simulink library "Library"  (R2018a)
settings: Solver=VariableStepAuto  StartTime=0.0  StopTime=10.0  RelTol=1e-3
values from neighbouring files (symbols this model uses):
  alpha = 1e-1*V_m^2    [dVOC.m]
  C_dc = 0.008*(n)    (= 1.6)    [VSM.m]    (also in dVOC.m; droop.m; droop_with_current_limitation.m; matching.m)
  C_f = n*300*10^-6    (= 0.06)    [VSM.m]    (also in dVOC.m; droop.m; droop_with_current_limitation.m; matching.m)
  D_p = (1/(m_p*w_b))    (= 101321.183642)    [VSM.m]
  droop_percentage = 1    [VSM.m]    (also in dVOC.m; droop.m; droop_with_current_limitation.m; matching.m)
  eta = m_p*V_m^2    [dVOC.m]
  eta_1 = w_b/Vdc_n    [VSM.m]    (also in dVOC.m; droop.m; droop_with_current_limitation.m; matching.m)
  i_ll = -1.15*(S_b/Vdc_n)-i_loss_dc    [VSM.m]    (also in dVOC.m; droop.m; droop_with_current_limitation.m; matching.m)
  i_ul = 1.15*(S_b/Vdc_n)+i_loss_dc    [VSM.m]    (also in dVOC.m; droop.m; droop_with_current_limitation.m; matching.m)
  J = D_p*tau_f    (= 2026.42367285)    [VSM.m]
  k_dc = eta_1/(Vdc_n*m_p)    [VSM.m]    (also in dVOC.m; droop.m; droop_with_current_limitation.m; matching.m)
  K_p = (1/Vdc_n)    [VSM.m]    (also in dVOC.m; droop.m; droop_with_current_limitation.m; matching.m)
  K_r = 1/R_dc    [VSM.m]    (also in dVOC.m; droop.m; droop_with_current_limitation.m; matching.m)
  Kff_i = 1    [VSM.m]    (also in dVOC.m; droop.m; droop_with_current_limitation.m; matching.m)
  Kff_v = 1    [VSM.m]    (also in dVOC.m; droop.m; droop_with_current_limitation.m; matching.m)
  Ki_i = (1/n)*1.19    (= 0.00595)    [VSM.m]    (also in dVOC.m; droop.m; droop_with_current_limitation.m; matching.m)
  Ki_v = (n)*1.161022    (= 232.2044)    [VSM.m]    (also in dVOC.m; droop.m; droop_with_current_limitation.m; matching.m)
  ki_v_ac = 4*5.2500e-04    (= 0.0021)    [VSM.m]    (also in dVOC.m = 0.5; droop.m = 0.5; droop_with_current_limitation.m = 0.5; matching.m = 0.5)
  Kp_i = 0.738891    [VSM.m]    (also in dVOC.m; droop.m; droop_with_current_limitation.m; matching.m)
  Kp_v = 0.52    [VSM.m]    (also in dVOC.m; droop.m; droop_with_current_limitation.m; matching.m)
  kp_v_ac = 0.001    [VSM.m]    (also in dVOC.m; droop.m; droop_with_current_limitation.m; matching.m)
  L_f = (1/n)*200*10^-6    (= 1e-06)    [VSM.m]    (also in dVOC.m; droop.m; droop_with_current_limitation.m; matching.m)
  m_p = (2*pi*0.5)/(S_b)    (= 3.14159265359e-08)    [VSM.m]    (also in dVOC.m; droop.m; droop_with_current_limitation.m; matching.m)
  n = 200    [VSM.m]    (also in dVOC.m; droop.m; droop_with_current_limitation.m; matching.m)
  R_dc = (Vdc_n/(0.05*(S_b)/Vdc_n))    [VSM.m]    (also in dVOC.m; droop.m; droop_with_current_limitation.m; matching.m)
  R_f = 0.001/n    (= 5e-06)    [VSM.m]    (also in dVOC.m; droop.m; droop_with_current_limitation.m; matching.m)
  S_b = 100*(10^6)    (= 100000000)    [VSM.m]    (also in dVOC.m; droop.m; droop_with_current_limitation.m; matching.m)
  T_en = T_load-0.5    (= 24.5)    [VSM.m]    (also in dVOC.m; droop.m; droop_with_current_limitation.m; matching.m)
  tau_dc = 0.05    [VSM.m]    (also in dVOC.m; droop.m; droop_with_current_limitation.m; matching.m)
  tau_g = 5    [VSM.m]    (also in dVOC.m; droop.m; droop_with_current_limitation.m; matching.m)
  V2_rms = 13800    [VSM.m]    (also in dVOC.m; droop.m; droop_with_current_limitation.m; matching.m)
  V_m = sqrt(2/3)*V1_rms    [VSM.m]    (also in dVOC.m; droop.m; droop_with_current_limitation.m; matching.m)
  Vdc_n = 3*V_m    [VSM.m]    (also in dVOC.m; droop.m; droop_with_current_limitation.m; matching.m)
  w_b = 2*pi*f_b    (= 314.159265359)    [VSM.m]    (also in dVOC.m; droop.m; droop_with_current_limitation.m; matching.m)
  w_f = 2*pi*5    (= 31.4159265359)    [VSM.m]    (also in dVOC.m; droop.m; droop_with_current_limitation.m; matching.m)
undefined symbols (not defined in the file or in its folder): i_dc, k_v_ac
libraries: powerlib x107, powerlib_meascontrol x48, cstblocks x5, simulink x3, sps_avr x1
(part 1 of 2)
settings Model: Creator=TayyebiA  LastModifiedBy=TayyebiA

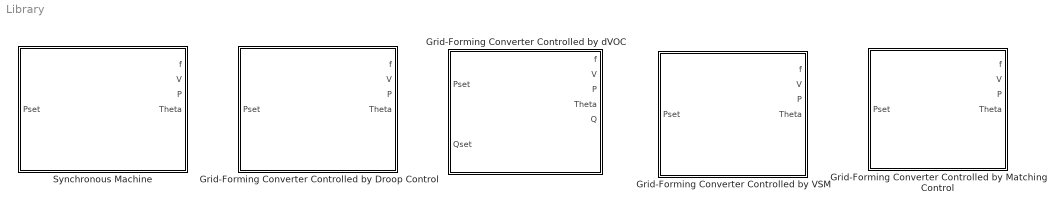
== system Library ==
  "Grid-Forming Converter Controlled by Droop Control " : Subsystem
  Grid-Forming Converter Controlled by Matching Control : Subsystem
  Grid-Forming Converter Controlled by VSM : Subsystem
  "Grid-Forming Converter Controlled by dVOC " : Subsystem
  Synchronous Machine : Subsystem

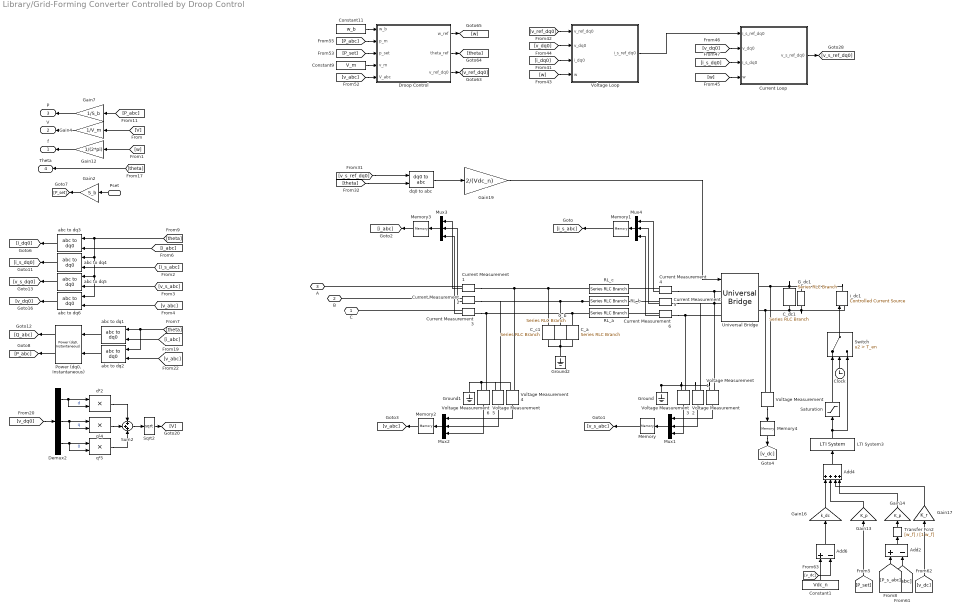
== system Library/Grid-Forming Converter Controlled by Droop Control  ==
  Pset : Inport
  Add2 : Sum  Inputs=+-
  Add4 : Sum  Inputs=++++
  Add6 : Sum  Inputs=+-
  C_a : powerlib/Elements/Series RLC Branch  LConnTagsString=__new0  RConnTagsString=__new0  BranchType=C  Resistance=1  Inductance=1e-3  SetiL0=off  InitialCurrent=0  Capacitance=C_f  Setx0=off  InitialVoltage=165  Measurements=None
  C_b : powerlib/Elements/Series RLC Branch  LConnTagsString=__new0  RConnTagsString=__new0  BranchType=C  Resistance=1  Inductance=1e-3  SetiL0=off  InitialCurrent=0  Capacitance=C_f  Setx0=off  InitialVoltage=165  Measurements=None
  C_c1 : powerlib/Elements/Series RLC Branch  LConnTagsString=__new0  RConnTagsString=__new0  BranchType=C  Resistance=1  Inductance=1e-3  SetiL0=off  InitialCurrent=0  Capacitance=C_f  Setx0=off  InitialVoltage=165  Measurements=None
  C_dc1 : powerlib/Elements/Series RLC Branch  LConnTagsString=__new0  RConnTagsString=__new0  BranchType=C  Resistance=1  Inductance=1e-3  SetiL0=off  InitialCurrent=0  Capacitance=C_dc  Setx0=off  InitialVoltage=Vdc_n  Measurements=None
  Clock : Clock
  Constant1 : Constant  Value=Vdc_n
  Constant11 : Constant  Value=w_b
  Constant9 : Constant  Value=V_m
  Current Loop : Subsystem
  Current Measurement{1..6} (6 alike) : powerlib/Measurements/Current Measurement  PhasorSimulation=off  OutputType=Complex  PSBequivalent=0
  Demux2 : Demux  Outputs=3
  Droop Control : Subsystem
  G_dc1 : powerlib/Elements/Series RLC Branch  LConnTagsString=__new0  RConnTagsString=__new0  BranchType=R  Resistance=R_dc  Inductance=1e-3  SetiL0=off  InitialCurrent=0  Capacitance=1e-6  Setx0=off  InitialVoltage=0  Measurements=None
  Gain12 : Gain  Gain=1/(2*pi)
  Gain13 : Gain  Gain=K_p
  Gain14 : Gain  Gain=K_p
  Gain16 : Gain  Gain=k_dc
  Gain17 : Gain  Gain=K_r
  Gain19 : Gain  Gain=2/(Vdc_n)
  Gain2 : Gain  Gain=S_b
  Gain4 : Gain  Gain=1/V_m
  Gain7 : Gain  Gain=1/S_b
  Ground : powerlib/Elements/Ground  LConnTagsString=a
  Ground1 : powerlib/Elements/Ground  LConnTagsString=a
  Ground2 : powerlib/Elements/Ground  LConnTagsString=a
  LTI System3 : cstblocks/LTI System  sys=tf(1,[tau_dc 1])  IC=[]
  Memory{,1..4} (5 alike) : Memory
  Mux{1..4} (4 alike) : Mux  Inputs=3
  "Power (dq0, Instantaneous)" : powerlib_meascontrol/Measurements/Power (dq0, Instantaneous)
      settings: SourceProductName=Simscape Power Systems  SourceProductBaseCode=PS
  RL_a : powerlib/Elements/Series RLC Branch  LConnTagsString=__new0  RConnTagsString=__new0  BranchType=RL  Resistance=R_f  Inductance=L_f  SetiL0=off  InitialCurrent=0  Capacitance=1e-6  Setx0=off  InitialVoltage=0  Measurements=Branch voltage and current
  RL_b : powerlib/Elements/Series RLC Branch  LConnTagsString=__new0  RConnTagsString=__new0  BranchType=RL  Resistance=R_f  Inductance=L_f  SetiL0=off  InitialCurrent=0  Capacitance=1e-6  Setx0=off  InitialVoltage=0  Measurements=None
  RL_c : powerlib/Elements/Series RLC Branch  LConnTagsString=__new0  RConnTagsString=__new0  BranchType=RL  Resistance=R_f  Inductance=L_f  SetiL0=off  InitialCurrent=0  Capacitance=1e-6  Setx0=off  InitialVoltage=0  Measurements=None
  Saturation : Saturate  UpperLimit=i_ul  LowerLimit=i_ll
  Sqrt2 : Sqrt  SaturateOnIntegerOverflow=on
  Sum2 : Sum  Inputs=+++  SaturateOnIntegerOverflow=on  InputSameDT=on  OutDataTypeStr=Inherit: Same as first input
  Switch : Switch  Criteria=u2 > Threshold  Threshold=T_en
  Transfer Fcn2 : TransferFcn  Numerator=[w_f]  Denominator=[1 w_f]
  Universal Bridge : powerlib/Power Electronics/Universal Bridge  Arms=3  SnubberResistance=1e5  SnubberCapacitance=inf  Device=Average-model based VSC  Ron=1e-3  Lon=0  ForwardVoltages="[  0  0  ]"  ForwardVoltage=0  GTOparameters=[ 10e-6 , 20e-6 ]  IGBTparameters=[ 1e-6 , 2e-6 ]  Measurements=None  Measurements_2=None  converterType=Rectifier
  Voltage Loop : Subsystem
  Voltage Measurement{,1..6} (7 alike) : powerlib/Measurements/Voltage Measurement  PhasorSimulation=off  OutputType=Complex  PSBequivalent=0
  abc to dq{1..6} (6 alike) : powerlib_meascontrol/Transformations/abc to dq0  Alignment=90 degrees behind phase A axis
  dq0 to abc : powerlib_meascontrol/Transformations/dq0 to abc  Alignment=90 degrees behind phase A axis
  d²2 : Product  SaturateOnIntegerOverflow=on  RndMeth=Zero  InputSameDT=on  OutDataTypeStr=Inherit: Same as first input
  i_dc1 : powerlib/Electrical Sources/Controlled Current Source  Initialize=off  Source_Type=DC  Amplitude=i_dc  Phase=0  Frequency=0  Measurements=None
  q²4 : Product  SaturateOnIntegerOverflow=on  RndMeth=Zero  InputSameDT=on  OutDataTypeStr=Inherit: Same as first input
  q²5 : Product  SaturateOnIntegerOverflow=on  RndMeth=Zero  InputSameDT=on  OutDataTypeStr=Inherit: Same as first input
  C : PMIOPort  Side=Right
  B : PMIOPort  Port=2  Side=Right
  A : PMIOPort  Port=3  Side=Right
  f : Outport
  V : Outport  Port=2
  P : Outport  Port=3
  Theta : Outport  Port=4
  wires:
  Add4/1 -> LTI System3/1
  Clock/1 -> Switch/2
  Saturation/1 -> Switch/1
  LTI System3/1 -> Switch/3, Saturation/1
  Gain7/1 -> P/1
  [P_abc] -> Gain7/1
  Current Measurement6/1 -> Mux4/3
  Current Measurement5/1 -> Mux4/2
  Current Measurement4/1 -> Mux4/1
  Current Measurement3/1 -> Mux3/3
  Current Measurement2/1 -> Mux3/2
  Current Measurement1/1 -> Mux3/1
  Voltage Measurement4/1 -> Mux2/1
  Voltage Measurement5/1 -> Mux2/2
  Voltage Measurement6/1 -> Mux2/3
  Voltage Measurement3/1 -> Mux1/3
  Voltage Measurement2/1 -> Mux1/2
  Voltage Measurement1/1 -> Mux1/1
  [V] -> Gain4/1
  Gain2/1 -> [P_set]
  Pset/1 -> Gain2/1
  Gain12/1 -> f/1
  [w] -> Gain12/1
  Mux2/1 -> Memory2/1
  Mux3/1 -> Memory3/1
  Mux1/1 -> Memory/1
  abc to dq1/1 -> "Power (dq0, Instantaneous)"/2
  abc to dq2/1 -> "Power (dq0, Instantaneous)"/1
  [theta] -> abc to dq2/2, abc to dq1/2
  [v_abc] -> abc to dq2/1
  "Power (dq0, Instantaneous)"/2 -> [Q_abc]
  "Power (dq0, Instantaneous)"/1 -> [P_abc]
  [i_abc] -> abc to dq1/1
  Gain4/1 -> V/1
  [theta] -> Theta/1
  [i_abc] -> abc to dq3/1
  [i_s_abc] -> abc to dq4/1
  [v_abc] -> abc to dq6/1
  [v_s_abc] -> abc to dq5/1
  [theta] -> abc to dq4/2, abc to dq5/2, abc to dq6/2, abc to dq3/2
  abc to dq3/1 -> [i_dq0]
  abc to dq4/1 -> [i_s_dq0]
  abc to dq5/1 -> [v_s_dq0]
  abc to dq6/1 -> [v_dq0]
  [theta] -> dq0 to abc/2
  q²4/1 -> Sum2/2
  [v_dq0] -> Demux2/1
  q²5/1 -> Sum2/3
  Sum2/1 -> Sqrt2/1
  Demux2/3 -> q²5/1, q²5/2  "0"
  d²2/1 -> Sum2/1
  Demux2/2 -> q²4/1, q²4/2  "q"
  Demux2/1 -> d²2/1, d²2/2  "d"
  Sqrt2/1 -> [V]
  Mux4/1 -> Memory1/1
  Memory2/1 -> [v_abc]
  Memory3/1 -> [i_abc]
  Voltage Measurement/1 -> Memory4/1
  Memory4/1 -> [v_dc]
  Memory/1 -> [v_s_abc]
  Memory1/1 -> [i_s_abc]
  dq0 to abc/1 -> Gain19/1
  [w] -> Current Loop/4(w)
  [v_ref_dq0] -> Voltage Loop/1(v_ref_dq0)
  [i_dq0] -> Voltage Loop/3(i_dq0)
  Voltage Loop/1(i_s_ref_dq0) -> Current Loop/1(i_s_ref_dq0)
  [v_dq0] -> Current Loop/2(v_dq0)
  [i_s_dq0] -> Current Loop/3(i_s_dq0)
  Current Loop/1(v_s_ref_dq0) -> [v_s_ref_dq0]
  [w] -> Voltage Loop/4(w)
  [v_dq0] -> Voltage Loop/2(v_dq0)
  Switch/1 -> i_dc1/1
  Gain19/1 -> Universal Bridge/1
  [v_s_ref_dq0] -> dq0 to abc/1
  Constant11/1 -> Droop Control/1(w_b)
  Droop Control/3(v_ref_dq0) -> [v_ref_dq0]
  [P_abc] -> Droop Control/2(p_m)
  Constant9/1 -> Droop Control/4(v_m)
  [v_abc] -> Droop Control/5(V_abc)
  Droop Control/2(theta_ref) -> [theta]
  Droop Control/1(w_ref) -> [w]
  [P_set] -> Droop Control/3(p_set)
  [P_abc] -> Add2/2
  Gain14/1 -> Add4/4
  [P_set] -> Gain13/1
  Gain13/1 -> Add4/2
  Gain16/1 -> Add4/1
  Constant1/1 -> Add6/1
  Gain17/1 -> Add4/3
  Add2/1 -> Transfer Fcn2/1
  Transfer Fcn2/1 -> Gain14/1
  [v_dc] -> Add6/2
  Add6/1 -> Gain16/1
  [P_s_abc] -> Add2/1
  [v_dc] -> Gain17/1
  connections:
  RL_b/RConn1 -- Voltage Measurement5/LConn1 -- Current Measurement2/LConn1 -- C_b/LConn1
  Voltage Measurement6/LConn1 -- Current Measurement3/LConn1 -- C_a/LConn1 -- RL_a/RConn1
  Current Measurement4/RConn1 -- RL_c/LConn1
  Current Measurement6/RConn1 -- RL_a/LConn1
  Current Measurement5/RConn1 -- RL_b/LConn1
  Voltage Measurement/LConn1 -- Universal Bridge/RConn1 -- C_dc1/LConn1 -- G_dc1/LConn1 -- i_dc1/RConn1
  Voltage Measurement6/LConn2 -- Voltage Measurement5/LConn2 -- Voltage Measurement4/LConn2 -- Ground1/LConn1
  Ground/LConn1 -- Voltage Measurement2/LConn2 -- Voltage Measurement1/LConn2 -- Voltage Measurement3/LConn2
  Current Measurement3/RConn1 -- C/RConn1
  Current Measurement2/RConn1 -- B/RConn1
  Current Measurement1/RConn1 -- A/RConn1
  Current Measurement6/LConn1 -- Universal Bridge/LConn3 -- Voltage Measurement3/LConn1
  Universal Bridge/LConn2 -- Current Measurement5/LConn1 -- Voltage Measurement2/LConn1
  Universal Bridge/LConn1 -- Current Measurement4/LConn1 -- Voltage Measurement1/LConn1
  Universal Bridge/RConn2 -- Voltage Measurement/LConn2 -- C_dc1/RConn1 -- G_dc1/RConn1 -- i_dc1/LConn1
  C_b/RConn1 -- C_a/RConn1 -- Ground2/LConn1 -- C_c1/RConn1
  Voltage Measurement4/LConn1 -- Current Measurement1/LConn1 -- C_c1/LConn1 -- RL_c/RConn1

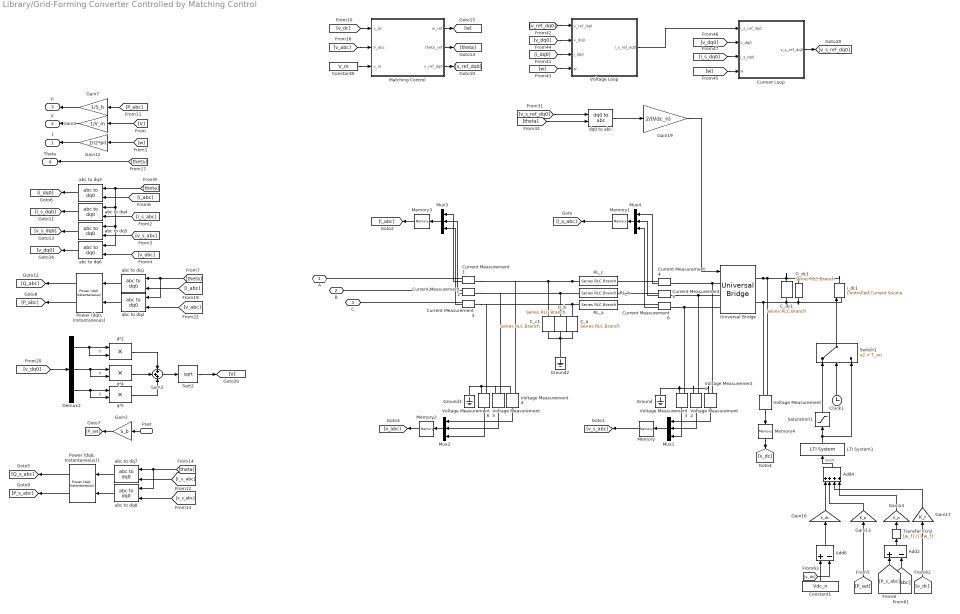
== system Library/Grid-Forming Converter Controlled by Matching Control ==
  Pset : Inport
  Add2 : Sum  Inputs=+-
  Add4 : Sum  Inputs=++++
  Add6 : Sum  Inputs=+-
  C_a : powerlib/Elements/Series RLC Branch  LConnTagsString=__new0  RConnTagsString=__new0  BranchType=C  Resistance=1  Inductance=1e-3  SetiL0=off  InitialCurrent=0  Capacitance=C_f  Setx0=off  InitialVoltage=165  Measurements=None
  C_b : powerlib/Elements/Series RLC Branch  LConnTagsString=__new0  RConnTagsString=__new0  BranchType=C  Resistance=1  Inductance=1e-3  SetiL0=off  InitialCurrent=0  Capacitance=C_f  Setx0=off  InitialVoltage=165  Measurements=None
  C_c1 : powerlib/Elements/Series RLC Branch  LConnTagsString=__new0  RConnTagsString=__new0  BranchType=C  Resistance=1  Inductance=1e-3  SetiL0=off  InitialCurrent=0  Capacitance=C_f  Setx0=off  InitialVoltage=165  Measurements=None
  C_dc1 : powerlib/Elements/Series RLC Branch  LConnTagsString=__new0  RConnTagsString=__new0  BranchType=C  Resistance=1  Inductance=1e-3  SetiL0=off  InitialCurrent=0  Capacitance=C_dc  Setx0=off  InitialVoltage=Vdc_n  Measurements=None
  Clock1 : Clock
  Constant1 : Constant  Value=Vdc_n
  Constant8 : Constant  Value=V_m
  Current Loop : Subsystem
  Current Measurement{1..6} (6 alike) : powerlib/Measurements/Current Measurement  PhasorSimulation=off  OutputType=Complex  PSBequivalent=0
  Demux2 : Demux  Outputs=3
  G_dc1 : powerlib/Elements/Series RLC Branch  LConnTagsString=__new0  RConnTagsString=__new0  BranchType=R  Resistance=R_dc  Inductance=1e-3  SetiL0=off  InitialCurrent=0  Capacitance=1e-6  Setx0=off  InitialVoltage=0  Measurements=None
  Gain12 : Gain  Gain=1/(2*pi)
  Gain13 : Gain  Gain=K_p
  Gain14 : Gain  Gain=K_p
  Gain16 : Gain  Gain=k_dc
  Gain17 : Gain  Gain=K_r
  Gain19 : Gain  Gain=2/(Vdc_n)
  Gain2 : Gain  Gain=S_b
  Gain4 : Gain  Gain=1/V_m
  Gain7 : Gain  Gain=1/S_b
  Ground : powerlib/Elements/Ground  LConnTagsString=a
  Ground1 : powerlib/Elements/Ground  LConnTagsString=a
  Ground2 : powerlib/Elements/Ground  LConnTagsString=a
  LTI System1 : cstblocks/LTI System  sys=tf(1,[tau_dc 1])  IC=[]
  Matching Control : Subsystem
  Memory{,1..4} (5 alike) : Memory
  Mux{1..4} (4 alike) : Mux  Inputs=3
  "Power (dq0, Instantaneous)" : powerlib_meascontrol/Measurements/Power (dq0, Instantaneous)
      settings: SourceProductName=Simscape Power Systems  SourceProductBaseCode=PS
  "Power (dq0, Instantaneous)1" : powerlib_meascontrol/Measurements/Power (dq0, Instantaneous)
      settings: SourceProductName=Simscape Power Systems  SourceProductBaseCode=PS
  RL_a : powerlib/Elements/Series RLC Branch  LConnTagsString=__new0  RConnTagsString=__new0  BranchType=RL  Resistance=R_f  Inductance=L_f  SetiL0=off  InitialCurrent=0  Capacitance=1e-6  Setx0=off  InitialVoltage=0  Measurements=Branch voltage and current
  RL_b : powerlib/Elements/Series RLC Branch  LConnTagsString=__new0  RConnTagsString=__new0  BranchType=RL  Resistance=R_f  Inductance=L_f  SetiL0=off  InitialCurrent=0  Capacitance=1e-6  Setx0=off  InitialVoltage=0  Measurements=None
  RL_c : powerlib/Elements/Series RLC Branch  LConnTagsString=__new0  RConnTagsString=__new0  BranchType=RL  Resistance=R_f  Inductance=L_f  SetiL0=off  InitialCurrent=0  Capacitance=1e-6  Setx0=off  InitialVoltage=0  Measurements=None
  Saturation1 : Saturate  UpperLimit=i_ul  LowerLimit=i_ll
  Sqrt2 : Sqrt  SaturateOnIntegerOverflow=on
  Sum2 : Sum  Inputs=+++  SaturateOnIntegerOverflow=on  InputSameDT=on  OutDataTypeStr=Inherit: Same as first input
  Switch1 : Switch  Criteria=u2 > Threshold  Threshold=T_en
  Transfer Fcn2 : TransferFcn  Numerator=[w_f]  Denominator=[1 w_f]
  Universal Bridge : powerlib/Power Electronics/Universal Bridge  Arms=3  SnubberResistance=1e5  SnubberCapacitance=inf  Device=Average-model based VSC  Ron=1e-3  Lon=0  ForwardVoltages="[  0  0  ]"  ForwardVoltage=0  GTOparameters=[ 10e-6 , 20e-6 ]  IGBTparameters=[ 1e-6 , 2e-6 ]  Measurements=None  Measurements_2=None  converterType=Rectifier
  Voltage Loop : Subsystem
  Voltage Measurement{,1..6} (7 alike) : powerlib/Measurements/Voltage Measurement  PhasorSimulation=off  OutputType=Complex  PSBequivalent=0
  abc to dq{1..8} (8 alike) : powerlib_meascontrol/Transformations/abc to dq0  Alignment=90 degrees behind phase A axis
  dq0 to abc : powerlib_meascontrol/Transformations/dq0 to abc  Alignment=90 degrees behind phase A axis
  d²2 : Product  SaturateOnIntegerOverflow=on  RndMeth=Zero  InputSameDT=on  OutDataTypeStr=Inherit: Same as first input
  i_dc1 : powerlib/Electrical Sources/Controlled Current Source  Initialize=off  Source_Type=DC  Amplitude=i_dc  Phase=0  Frequency=0  Measurements=None
  q²4 : Product  SaturateOnIntegerOverflow=on  RndMeth=Zero  InputSameDT=on  OutDataTypeStr=Inherit: Same as first input
  q²5 : Product  SaturateOnIntegerOverflow=on  RndMeth=Zero  InputSameDT=on  OutDataTypeStr=Inherit: Same as first input
  A : PMIOPort  Side=Right
  B : PMIOPort  Port=2  Side=Right
  C : PMIOPort  Port=3  Side=Right
  f : Outport
  V : Outport  Port=2
  P : Outport  Port=3
  Theta : Outport  Port=4
  wires:
  [v_s_ref_dq0] -> dq0 to abc/1
  Gain19/1 -> Universal Bridge/1
  Switch1/1 -> i_dc1/1
  [v_dq0] -> Voltage Loop/2(v_dq0)
  [w] -> Voltage Loop/4(w)
  Current Loop/1(v_s_ref_dq0) -> [v_s_ref_dq0]
  [i_s_dq0] -> Current Loop/3(i_s_dq0)
  [v_dq0] -> Current Loop/2(v_dq0)
  Voltage Loop/1(i_s_ref_dq0) -> Current Loop/1(i_s_ref_dq0)
  [i_dq0] -> Voltage Loop/3(i_dq0)
  [v_ref_dq0] -> Voltage Loop/1(v_ref_dq0)
  [w] -> Current Loop/4(w)
  dq0 to abc/1 -> Gain19/1
  Memory1/1 -> [i_s_abc]
  Memory/1 -> [v_s_abc]
  Memory4/1 -> [v_dc]
  Voltage Measurement/1 -> Memory4/1
  Memory3/1 -> [i_abc]
  Memory2/1 -> [v_abc]
  Mux4/1 -> Memory1/1
  Sqrt2/1 -> [V]
  Demux2/1 -> d²2/2, d²2/1  "d"
  Demux2/2 -> q²4/2, q²4/1  "q"
  d²2/1 -> Sum2/1
  Demux2/3 -> q²5/2, q²5/1  "0"
  Sum2/1 -> Sqrt2/1
  q²5/1 -> Sum2/3
  [v_dq0] -> Demux2/1
  q²4/1 -> Sum2/2
  [theta] -> dq0 to abc/2
  abc to dq6/1 -> [v_dq0]
  abc to dq5/1 -> [v_s_dq0]
  abc to dq4/1 -> [i_s_dq0]
  abc to dq3/1 -> [i_dq0]
  [theta] -> abc to dq3/2, abc to dq6/2, abc to dq5/2, abc to dq4/2
  [v_s_abc] -> abc to dq5/1
  [v_abc] -> abc to dq6/1
  [i_s_abc] -> abc to dq4/1
  [i_abc] -> abc to dq3/1
  [theta] -> Theta/1
  Gain4/1 -> V/1
  [i_abc] -> abc to dq1/1
  "Power (dq0, Instantaneous)"/1 -> [P_abc]
  "Power (dq0, Instantaneous)"/2 -> [Q_abc]
  [v_abc] -> abc to dq2/1
  [theta] -> abc to dq1/2, abc to dq2/2
  abc to dq2/1 -> "Power (dq0, Instantaneous)"/1
  abc to dq1/1 -> "Power (dq0, Instantaneous)"/2
  Mux1/1 -> Memory/1
  Mux3/1 -> Memory3/1
  Mux2/1 -> Memory2/1
  [w] -> Gain12/1
  Gain12/1 -> f/1
  Pset/1 -> Gain2/1
  Gain2/1 -> [P_set]
  [V] -> Gain4/1
  Voltage Measurement1/1 -> Mux1/1
  Voltage Measurement2/1 -> Mux1/2
  Voltage Measurement3/1 -> Mux1/3
  Voltage Measurement6/1 -> Mux2/3
  Voltage Measurement5/1 -> Mux2/2
  Voltage Measurement4/1 -> Mux2/1
  Current Measurement1/1 -> Mux3/1
  Current Measurement2/1 -> Mux3/2
  Current Measurement3/1 -> Mux3/3
  Current Measurement4/1 -> Mux4/1
  Current Measurement5/1 -> Mux4/2
  Current Measurement6/1 -> Mux4/3
  [P_abc] -> Gain7/1
  Gain7/1 -> P/1
  [P_s_abc] -> Add2/1
  [v_dc] -> Gain17/1
  Gain17/1 -> Add4/3
  Constant1/1 -> Add6/1
  Clock1/1 -> Switch1/2
  [P_abc] -> Add2/2
  Add6/1 -> Gain16/1
  Add4/1 -> LTI System1/1  "input"
  [P_set] -> Gain13/1
  Gain14/1 -> Add4/4
  Saturation1/1 -> Switch1/1
  LTI System1/1 -> Saturation1/1, Switch1/3
  Gain16/1 -> Add4/1
  Constant8/1 -> Matching Control/3(v_m)
  Matching Control/3(v_ref_dq0) -> [v_ref_dq0]
  Matching Control/2(theta_ref) -> [theta]
  Gain13/1 -> Add4/2
  [v_dc] -> Matching Control/1(v_dc)
  [v_dc] -> Add6/2
  [v_abc] -> Matching Control/2(V_abc)
  Transfer Fcn2/1 -> Gain14/1
  Matching Control/1(w_ref) -> [w]
  Add2/1 -> Transfer Fcn2/1
  abc to dq8/1 -> "Power (dq0, Instantaneous)1"/1
  [i_s_abc] -> abc to dq7/1
  [v_s_abc] -> abc to dq8/1
  abc to dq7/1 -> "Power (dq0, Instantaneous)1"/2
  [theta] -> abc to dq7/2, abc to dq8/2
  "Power (dq0, Instantaneous)1"/2 -> [Q_s_abc]
  "Power (dq0, Instantaneous)1"/1 -> [P_s_abc]
  connections:
  RL_c/RConn1 -- C_c1/LConn1 -- Current Measurement1/LConn1 -- Voltage Measurement4/LConn1
  C_c1/RConn1 -- Ground2/LConn1 -- C_a/RConn1 -- C_b/RConn1
  Universal Bridge/RConn2 -- i_dc1/LConn1 -- G_dc1/RConn1 -- C_dc1/RConn1 -- Voltage Measurement/LConn2
  Voltage Measurement1/LConn1 -- Current Measurement4/LConn1 -- Universal Bridge/LConn1
  Voltage Measurement2/LConn1 -- Current Measurement5/LConn1 -- Universal Bridge/LConn2
  Voltage Measurement3/LConn1 -- Universal Bridge/LConn3 -- Current Measurement6/LConn1
  Current Measurement1/RConn1 -- A/RConn1
  Current Measurement2/RConn1 -- B/RConn1
  Current Measurement3/RConn1 -- C/RConn1
  Voltage Measurement3/LConn2 -- Voltage Measurement1/LConn2 -- Voltage Measurement2/LConn2 -- Ground/LConn1
  Ground1/LConn1 -- Voltage Measurement4/LConn2 -- Voltage Measurement5/LConn2 -- Voltage Measurement6/LConn2
  Universal Bridge/RConn1 -- Voltage Measurement/LConn1 -- i_dc1/RConn1 -- G_dc1/LConn1 -- C_dc1/LConn1
  Current Measurement5/RConn1 -- RL_b/LConn1
  Current Measurement6/RConn1 -- RL_a/LConn1
  Current Measurement4/RConn1 -- RL_c/LConn1
  RL_a/RConn1 -- C_a/LConn1 -- Current Measurement3/LConn1 -- Voltage Measurement6/LConn1
  C_b/LConn1 -- Current Measurement2/LConn1 -- Voltage Measurement5/LConn1 -- RL_b/RConn1

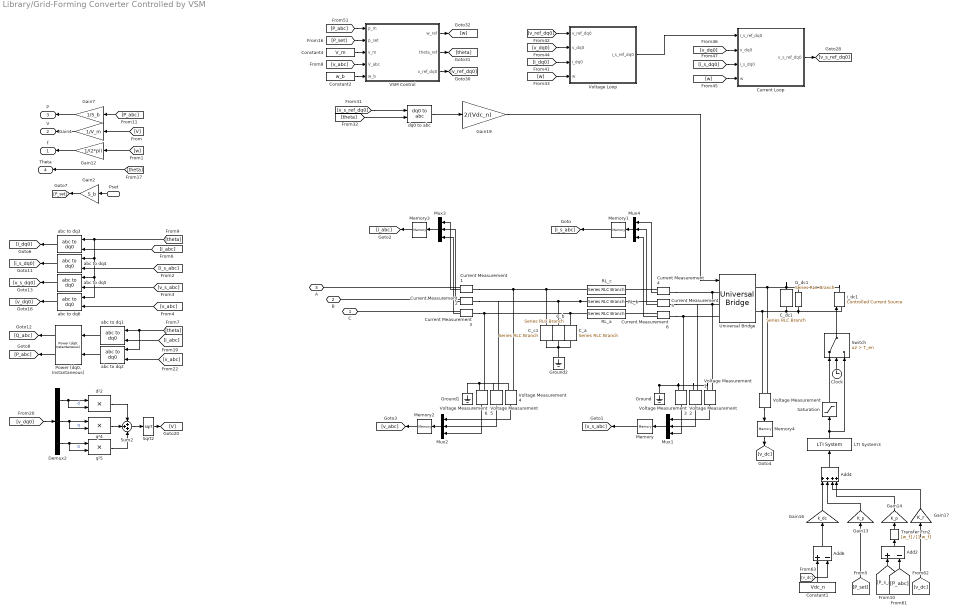
== system Library/Grid-Forming Converter Controlled by VSM ==
  Pset : Inport
  Add2 : Sum  Inputs=+-
  Add4 : Sum  Inputs=++++
  Add6 : Sum  Inputs=+-
  C_a : powerlib/Elements/Series RLC Branch  LConnTagsString=__new0  RConnTagsString=__new0  BranchType=C  Resistance=1  Inductance=1e-3  SetiL0=off  InitialCurrent=0  Capacitance=C_f  Setx0=off  InitialVoltage=165  Measurements=None
  C_b : powerlib/Elements/Series RLC Branch  LConnTagsString=__new0  RConnTagsString=__new0  BranchType=C  Resistance=1  Inductance=1e-3  SetiL0=off  InitialCurrent=0  Capacitance=C_f  Setx0=off  InitialVoltage=165  Measurements=None
  C_c1 : powerlib/Elements/Series RLC Branch  LConnTagsString=__new0  RConnTagsString=__new0  BranchType=C  Resistance=1  Inductance=1e-3  SetiL0=off  InitialCurrent=0  Capacitance=C_f  Setx0=off  InitialVoltage=165  Measurements=None
  C_dc1 : powerlib/Elements/Series RLC Branch  LConnTagsString=__new0  RConnTagsString=__new0  BranchType=C  Resistance=1  Inductance=1e-3  SetiL0=off  InitialCurrent=0  Capacitance=C_dc  Setx0=off  InitialVoltage=Vdc_n  Measurements=None
  Clock : Clock
  Constant1 : Constant  Value=Vdc_n
  Constant2 : Constant  Value=w_b
  Constant4 : Constant  Value=V_m
  Current Loop : Subsystem
  Current Measurement{1..6} (6 alike) : powerlib/Measurements/Current Measurement  PhasorSimulation=off  OutputType=Complex  PSBequivalent=0
  Demux2 : Demux  Outputs=3
  G_dc1 : powerlib/Elements/Series RLC Branch  LConnTagsString=__new0  RConnTagsString=__new0  BranchType=R  Resistance=R_dc  Inductance=1e-3  SetiL0=off  InitialCurrent=0  Capacitance=1e-6  Setx0=off  InitialVoltage=0  Measurements=None
  Gain12 : Gain  Gain=1/(2*pi)
  Gain13 : Gain  Gain=K_p
  Gain14 : Gain  Gain=K_p
  Gain16 : Gain  Gain=k_dc
  Gain17 : Gain  Gain=K_r
  Gain19 : Gain  Gain=2/(Vdc_n)
  Gain2 : Gain  Gain=S_b
  Gain4 : Gain  Gain=1/V_m
  Gain7 : Gain  Gain=1/S_b
  Ground : powerlib/Elements/Ground  LConnTagsString=a
  Ground1 : powerlib/Elements/Ground  LConnTagsString=a
  Ground2 : powerlib/Elements/Ground  LConnTagsString=a
  LTI System3 : cstblocks/LTI System  sys=tf(1,[tau_dc 1])  IC=[]
  Memory{,1..4} (5 alike) : Memory
  Mux{1..4} (4 alike) : Mux  Inputs=3
  "Power (dq0, Instantaneous)" : powerlib_meascontrol/Measurements/Power (dq0, Instantaneous)
      settings: SourceProductName=Simscape Power Systems  SourceProductBaseCode=PS
  RL_a : powerlib/Elements/Series RLC Branch  LConnTagsString=__new0  RConnTagsString=__new0  BranchType=RL  Resistance=R_f  Inductance=L_f  SetiL0=off  InitialCurrent=0  Capacitance=1e-6  Setx0=off  InitialVoltage=0  Measurements=Branch voltage and current
  RL_b : powerlib/Elements/Series RLC Branch  LConnTagsString=__new0  RConnTagsString=__new0  BranchType=RL  Resistance=R_f  Inductance=L_f  SetiL0=off  InitialCurrent=0  Capacitance=1e-6  Setx0=off  InitialVoltage=0  Measurements=None
  RL_c : powerlib/Elements/Series RLC Branch  LConnTagsString=__new0  RConnTagsString=__new0  BranchType=RL  Resistance=R_f  Inductance=L_f  SetiL0=off  InitialCurrent=0  Capacitance=1e-6  Setx0=off  InitialVoltage=0  Measurements=None
  Saturation : Saturate  UpperLimit=i_ul  LowerLimit=i_ll
  Sqrt2 : Sqrt  SaturateOnIntegerOverflow=on
  Sum2 : Sum  Inputs=+++  SaturateOnIntegerOverflow=on  InputSameDT=on  OutDataTypeStr=Inherit: Same as first input
  Switch : Switch  Criteria=u2 > Threshold  Threshold=T_en
  Transfer Fcn2 : TransferFcn  Numerator=[w_f]  Denominator=[1 w_f]
  Universal Bridge : powerlib/Power Electronics/Universal Bridge  Arms=3  SnubberResistance=1e5  SnubberCapacitance=inf  Device=Average-model based VSC  Ron=1e-3  Lon=0  ForwardVoltages="[  0  0  ]"  ForwardVoltage=0  GTOparameters=[ 10e-6 , 20e-6 ]  IGBTparameters=[ 1e-6 , 2e-6 ]  Measurements=None  Measurements_2=None  converterType=Rectifier
  VSM Control : Subsystem
  Voltage Loop : Subsystem
  Voltage Measurement{,1..6} (7 alike) : powerlib/Measurements/Voltage Measurement  PhasorSimulation=off  OutputType=Complex  PSBequivalent=0
  abc to dq{1..6} (6 alike) : powerlib_meascontrol/Transformations/abc to dq0  Alignment=90 degrees behind phase A axis
  dq0 to abc : powerlib_meascontrol/Transformations/dq0 to abc  Alignment=90 degrees behind phase A axis
  d²2 : Product  SaturateOnIntegerOverflow=on  RndMeth=Zero  InputSameDT=on  OutDataTypeStr=Inherit: Same as first input
  i_dc1 : powerlib/Electrical Sources/Controlled Current Source  Initialize=off  Source_Type=DC  Amplitude=i_dc  Phase=0  Frequency=0  Measurements=None
  q²4 : Product  SaturateOnIntegerOverflow=on  RndMeth=Zero  InputSameDT=on  OutDataTypeStr=Inherit: Same as first input
  q²5 : Product  SaturateOnIntegerOverflow=on  RndMeth=Zero  InputSameDT=on  OutDataTypeStr=Inherit: Same as first input
  C : PMIOPort  Side=Right
  B : PMIOPort  Port=2  Side=Right
  A : PMIOPort  Port=3  Side=Right
  f : Outport
  V : Outport  Port=2
  P : Outport  Port=3
  Theta : Outport  Port=4
  wires:
  Add4/1 -> LTI System3/1
  Clock/1 -> Switch/2
  Saturation/1 -> Switch/1
  LTI System3/1 -> Switch/3, Saturation/1
  Gain7/1 -> P/1
  [P_abc] -> Gain7/1
  Current Measurement6/1 -> Mux4/3
  Current Measurement5/1 -> Mux4/2
  Current Measurement4/1 -> Mux4/1
  Current Measurement3/1 -> Mux3/3
  Current Measurement2/1 -> Mux3/2
  Current Measurement1/1 -> Mux3/1
  Voltage Measurement4/1 -> Mux2/1
  Voltage Measurement5/1 -> Mux2/2
  Voltage Measurement6/1 -> Mux2/3
  Voltage Measurement3/1 -> Mux1/3
  Voltage Measurement2/1 -> Mux1/2
  Voltage Measurement1/1 -> Mux1/1
  [V] -> Gain4/1
  Gain2/1 -> [P_set]
  Pset/1 -> Gain2/1
  Gain12/1 -> f/1
  [w] -> Gain12/1
  Mux2/1 -> Memory2/1
  Mux3/1 -> Memory3/1
  Mux1/1 -> Memory/1
  abc to dq1/1 -> "Power (dq0, Instantaneous)"/2
  abc to dq2/1 -> "Power (dq0, Instantaneous)"/1
  [theta] -> abc to dq2/2, abc to dq1/2
  [v_abc] -> abc to dq2/1
  "Power (dq0, Instantaneous)"/2 -> [Q_abc]
  "Power (dq0, Instantaneous)"/1 -> [P_abc]
  [i_abc] -> abc to dq1/1
  Gain4/1 -> V/1
  [theta] -> Theta/1
  [i_abc] -> abc to dq3/1
  [i_s_abc] -> abc to dq4/1
  [v_abc] -> abc to dq6/1
  [v_s_abc] -> abc to dq5/1
  [theta] -> abc to dq4/2, abc to dq5/2, abc to dq6/2, abc to dq3/2
  abc to dq3/1 -> [i_dq0]
  abc to dq4/1 -> [i_s_dq0]
  abc to dq5/1 -> [v_s_dq0]
  abc to dq6/1 -> [v_dq0]
  [theta] -> dq0 to abc/2
  q²4/1 -> Sum2/2
  [v_dq0] -> Demux2/1
  q²5/1 -> Sum2/3
  Sum2/1 -> Sqrt2/1
  Demux2/3 -> q²5/1, q²5/2  "0"
  d²2/1 -> Sum2/1
  Demux2/2 -> q²4/1, q²4/2  "q"
  Demux2/1 -> d²2/1, d²2/2  "d"
  Sqrt2/1 -> [V]
  Mux4/1 -> Memory1/1
  Memory2/1 -> [v_abc]
  Memory3/1 -> [i_abc]
  Voltage Measurement/1 -> Memory4/1
  Memory4/1 -> [v_dc]
  Memory/1 -> [v_s_abc]
  Memory1/1 -> [i_s_abc]
  dq0 to abc/1 -> Gain19/1
  [w] -> Current Loop/4(w)
  [v_ref_dq0] -> Voltage Loop/1(v_ref_dq0)
  [i_dq0] -> Voltage Loop/3(i_dq0)
  Voltage Loop/1(i_s_ref_dq0) -> Current Loop/1(i_s_ref_dq0)
  [v_dq0] -> Current Loop/2(v_dq0)
  [i_s_dq0] -> Current Loop/3(i_s_dq0)
  Current Loop/1(v_s_ref_dq0) -> [v_s_ref_dq0]
  [w] -> Voltage Loop/4(w)
  [v_dq0] -> Voltage Loop/2(v_dq0)
  Switch/1 -> i_dc1/1
  Gain19/1 -> Universal Bridge/1
  [v_s_ref_dq0] -> dq0 to abc/1
  VSM Control/2(theta_ref) -> [theta]
  VSM Control/3(v_ref_dq0) -> [v_ref_dq0]
  Constant2/1 -> VSM Control/5(w_b)
  [P_set] -> VSM Control/2(p_set)
  [v_abc] -> VSM Control/4(V_abc)
  [P_abc] -> VSM Control/1(p_m)
  VSM Control/1(w_ref) -> [w]
  Constant4/1 -> VSM Control/3(v_m)
  [P_abc] -> Add2/2
  Gain14/1 -> Add4/4
  [P_set] -> Gain13/1
  Gain13/1 -> Add4/2
  Gain16/1 -> Add4/1
  Constant1/1 -> Add6/1
  Gain17/1 -> Add4/3
  Add2/1 -> Transfer Fcn2/1
  Transfer Fcn2/1 -> Gain14/1
  [v_dc] -> Add6/2
  Add6/1 -> Gain16/1
  [P_s_abc] -> Add2/1
  [v_dc] -> Gain17/1
  connections:
  RL_b/RConn1 -- Voltage Measurement5/LConn1 -- Current Measurement2/LConn1 -- C_b/LConn1
  Voltage Measurement6/LConn1 -- Current Measurement3/LConn1 -- C_a/LConn1 -- RL_a/RConn1
  Current Measurement4/RConn1 -- RL_c/LConn1
  Current Measurement6/RConn1 -- RL_a/LConn1
  Current Measurement5/RConn1 -- RL_b/LConn1
  Voltage Measurement/LConn1 -- Universal Bridge/RConn1 -- C_dc1/LConn1 -- G_dc1/LConn1 -- i_dc1/RConn1
  Voltage Measurement6/LConn2 -- Voltage Measurement5/LConn2 -- Voltage Measurement4/LConn2 -- Ground1/LConn1
  Ground/LConn1 -- Voltage Measurement2/LConn2 -- Voltage Measurement1/LConn2 -- Voltage Measurement3/LConn2
  Current Measurement3/RConn1 -- C/RConn1
  Current Measurement2/RConn1 -- B/RConn1
  Current Measurement1/RConn1 -- A/RConn1
  Current Measurement6/LConn1 -- Universal Bridge/LConn3 -- Voltage Measurement3/LConn1
  Universal Bridge/LConn2 -- Current Measurement5/LConn1 -- Voltage Measurement2/LConn1
  Universal Bridge/LConn1 -- Current Measurement4/LConn1 -- Voltage Measurement1/LConn1
  Universal Bridge/RConn2 -- Voltage Measurement/LConn2 -- C_dc1/RConn1 -- G_dc1/RConn1 -- i_dc1/LConn1
  C_b/RConn1 -- C_a/RConn1 -- Ground2/LConn1 -- C_c1/RConn1
  Voltage Measurement4/LConn1 -- Current Measurement1/LConn1 -- C_c1/LConn1 -- RL_c/RConn1

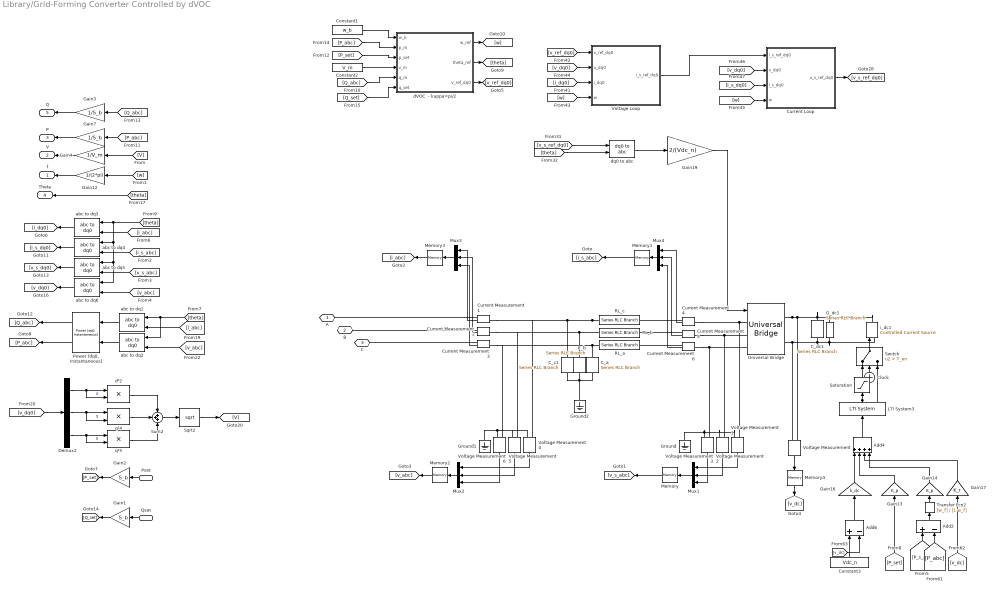
== system Library/Grid-Forming Converter Controlled by dVOC  ==
  Pset : Inport
  Qset : Inport  Port=2
  Add2 : Sum  Inputs=+-
  Add4 : Sum  Inputs=++++
  Add6 : Sum  Inputs=+-
  C_a : powerlib/Elements/Series RLC Branch  LConnTagsString=__new0  RConnTagsString=__new0  BranchType=C  Resistance=1  Inductance=1e-3  SetiL0=off  InitialCurrent=0  Capacitance=C_f  Setx0=off  InitialVoltage=165  Measurements=None
  C_b : powerlib/Elements/Series RLC Branch  LConnTagsString=__new0  RConnTagsString=__new0  BranchType=C  Resistance=1  Inductance=1e-3  SetiL0=off  InitialCurrent=0  Capacitance=C_f  Setx0=off  InitialVoltage=165  Measurements=None
  C_c1 : powerlib/Elements/Series RLC Branch  LConnTagsString=__new0  RConnTagsString=__new0  BranchType=C  Resistance=1  Inductance=1e-3  SetiL0=off  InitialCurrent=0  Capacitance=C_f  Setx0=off  InitialVoltage=165  Measurements=None
  C_dc1 : powerlib/Elements/Series RLC Branch  LConnTagsString=__new0  RConnTagsString=__new0  BranchType=C  Resistance=1  Inductance=1e-3  SetiL0=off  InitialCurrent=0  Capacitance=C_dc  Setx0=off  InitialVoltage=Vdc_n  Measurements=None
  Clock : Clock
  Constant1 : Constant  Value=w_b
  Constant2 : Constant  Value=V_m
  Constant3 : Constant  Value=Vdc_n
  Current Loop : Subsystem
  Current Measurement{1..6} (6 alike) : powerlib/Measurements/Current Measurement  PhasorSimulation=off  OutputType=Complex  PSBequivalent=0
  Demux2 : Demux  Outputs=3
  G_dc1 : powerlib/Elements/Series RLC Branch  LConnTagsString=__new0  RConnTagsString=__new0  BranchType=R  Resistance=R_dc  Inductance=1e-3  SetiL0=off  InitialCurrent=0  Capacitance=1e-6  Setx0=off  InitialVoltage=0  Measurements=None
  Gain1 : Gain  Gain=S_b
  Gain12 : Gain  Gain=1/(2*pi)
  Gain13 : Gain  Gain=K_p
  Gain14 : Gain  Gain=K_p
  Gain16 : Gain  Gain=k_dc
  Gain17 : Gain  Gain=K_r
  Gain19 : Gain  Gain=2/(Vdc_n)
  Gain2 : Gain  Gain=S_b
  Gain3 : Gain  Gain=1/S_b
  Gain4 : Gain  Gain=1/V_m
  Gain7 : Gain  Gain=1/S_b
  Ground : powerlib/Elements/Ground  LConnTagsString=a
  Ground1 : powerlib/Elements/Ground  LConnTagsString=a
  Ground2 : powerlib/Elements/Ground  LConnTagsString=a
  LTI System3 : cstblocks/LTI System  sys=tf(1,[tau_dc 1])  IC=[]
  Memory{,1..4} (5 alike) : Memory
  Mux{1..4} (4 alike) : Mux  Inputs=3
  "Power (dq0, Instantaneous)" : powerlib_meascontrol/Measurements/Power (dq0, Instantaneous)
      settings: SourceProductName=Simscape Power Systems  SourceProductBaseCode=PS
  RL_a : powerlib/Elements/Series RLC Branch  LConnTagsString=__new0  RConnTagsString=__new0  BranchType=RL  Resistance=R_f  Inductance=L_f  SetiL0=off  InitialCurrent=0  Capacitance=1e-6  Setx0=off  InitialVoltage=0  Measurements=Branch voltage and current
  RL_b : powerlib/Elements/Series RLC Branch  LConnTagsString=__new0  RConnTagsString=__new0  BranchType=RL  Resistance=R_f  Inductance=L_f  SetiL0=off  InitialCurrent=0  Capacitance=1e-6  Setx0=off  InitialVoltage=0  Measurements=None
  RL_c : powerlib/Elements/Series RLC Branch  LConnTagsString=__new0  RConnTagsString=__new0  BranchType=RL  Resistance=R_f  Inductance=L_f  SetiL0=off  InitialCurrent=0  Capacitance=1e-6  Setx0=off  InitialVoltage=0  Measurements=None
  Saturation : Saturate  UpperLimit=i_ul  LowerLimit=i_ll
  Sqrt2 : Sqrt  SaturateOnIntegerOverflow=on
  Sum2 : Sum  Inputs=+++  SaturateOnIntegerOverflow=on  InputSameDT=on  OutDataTypeStr=Inherit: Same as first input
  Switch : Switch  Criteria=u2 > Threshold  Threshold=T_en
  Transfer Fcn2 : TransferFcn  Numerator=[w_f]  Denominator=[1 w_f]
  Universal Bridge : powerlib/Power Electronics/Universal Bridge  Arms=3  SnubberResistance=1e5  SnubberCapacitance=inf  Device=Average-model based VSC  Ron=1e-3  Lon=0  ForwardVoltages="[  0  0  ]"  ForwardVoltage=0  GTOparameters=[ 10e-6 , 20e-6 ]  IGBTparameters=[ 1e-6 , 2e-6 ]  Measurements=None  Measurements_2=None  converterType=Rectifier
  Voltage Loop : Subsystem
  Voltage Measurement{,1..6} (7 alike) : powerlib/Measurements/Voltage Measurement  PhasorSimulation=off  OutputType=Complex  PSBequivalent=0
  abc to dq{1..6} (6 alike) : powerlib_meascontrol/Transformations/abc to dq0  Alignment=90 degrees behind phase A axis
  dVOC  - kappa=pi/2 : Subsystem
  dq0 to abc : powerlib_meascontrol/Transformations/dq0 to abc  Alignment=90 degrees behind phase A axis
  d²2 : Product  SaturateOnIntegerOverflow=on  RndMeth=Zero  InputSameDT=on  OutDataTypeStr=Inherit: Same as first input
  i_dc1 : powerlib/Electrical Sources/Controlled Current Source  Initialize=off  Source_Type=DC  Amplitude=i_dc  Phase=0  Frequency=0  Measurements=None
  q²4 : Product  SaturateOnIntegerOverflow=on  RndMeth=Zero  InputSameDT=on  OutDataTypeStr=Inherit: Same as first input
  q²5 : Product  SaturateOnIntegerOverflow=on  RndMeth=Zero  InputSameDT=on  OutDataTypeStr=Inherit: Same as first input
  A : PMIOPort  Side=Right
  B : PMIOPort  Port=2  Side=Right
  C : PMIOPort  Port=3  Side=Right
  f : Outport
  V : Outport  Port=2
  P : Outport  Port=3
  Theta : Outport  Port=4
  Q : Outport  Port=5
  wires:
  [v_s_ref_dq0] -> dq0 to abc/1
  Gain19/1 -> Universal Bridge/1
  Switch/1 -> i_dc1/1
  [v_dq0] -> Voltage Loop/2(v_dq0)
  [w] -> Voltage Loop/4(w)
  Current Loop/1(v_s_ref_dq0) -> [v_s_ref_dq0]
  [i_s_dq0] -> Current Loop/3(i_s_dq0)
  [v_dq0] -> Current Loop/2(v_dq0)
  Voltage Loop/1(i_s_ref_dq0) -> Current Loop/1(i_s_ref_dq0)
  [i_dq0] -> Voltage Loop/3(i_dq0)
  [v_ref_dq0] -> Voltage Loop/1(v_ref_dq0)
  [w] -> Current Loop/4(w)
  dq0 to abc/1 -> Gain19/1
  Memory1/1 -> [i_s_abc]
  Memory/1 -> [v_s_abc]
  Memory4/1 -> [v_dc]
  Voltage Measurement/1 -> Memory4/1
  Memory3/1 -> [i_abc]
  Memory2/1 -> [v_abc]
  Mux4/1 -> Memory1/1
  Sqrt2/1 -> [V]
  Demux2/1 -> d²2/2, d²2/1  "d"
  Demux2/2 -> q²4/2, q²4/1  "q"
  d²2/1 -> Sum2/1
  Demux2/3 -> q²5/2, q²5/1  "0"
  Sum2/1 -> Sqrt2/1
  q²5/1 -> Sum2/3
  [v_dq0] -> Demux2/1
  q²4/1 -> Sum2/2
  [theta] -> dq0 to abc/2
  abc to dq6/1 -> [v_dq0]
  abc to dq5/1 -> [v_s_dq0]
  abc to dq4/1 -> [i_s_dq0]
  abc to dq3/1 -> [i_dq0]
  [theta] -> abc to dq3/2, abc to dq6/2, abc to dq5/2, abc to dq4/2
  [v_s_abc] -> abc to dq5/1
  [v_abc] -> abc to dq6/1
  [i_s_abc] -> abc to dq4/1
  [i_abc] -> abc to dq3/1
  [theta] -> Theta/1
  Gain4/1 -> V/1
  [i_abc] -> abc to dq1/1
  "Power (dq0, Instantaneous)"/1 -> [P_abc]
  "Power (dq0, Instantaneous)"/2 -> [Q_abc]
  [v_abc] -> abc to dq2/1
  [theta] -> abc to dq1/2, abc to dq2/2
  abc to dq2/1 -> "Power (dq0, Instantaneous)"/1
  abc to dq1/1 -> "Power (dq0, Instantaneous)"/2
  Mux1/1 -> Memory/1
  Mux3/1 -> Memory3/1
  Mux2/1 -> Memory2/1
  [w] -> Gain12/1
  Gain12/1 -> f/1
  Pset/1 -> Gain2/1
  Gain2/1 -> [P_set]
  [V] -> Gain4/1
  Voltage Measurement1/1 -> Mux1/1
  Voltage Measurement2/1 -> Mux1/2
  Voltage Measurement3/1 -> Mux1/3
  Voltage Measurement6/1 -> Mux2/3
  Voltage Measurement5/1 -> Mux2/2
  Voltage Measurement4/1 -> Mux2/1
  Current Measurement1/1 -> Mux3/1
  Current Measurement2/1 -> Mux3/2
  Current Measurement3/1 -> Mux3/3
  Current Measurement4/1 -> Mux4/1
  Current Measurement5/1 -> Mux4/2
  Current Measurement6/1 -> Mux4/3
  [P_abc] -> Gain7/1
  Gain7/1 -> P/1
  LTI System3/1 -> Switch/3, Saturation/1
  Saturation/1 -> Switch/1
  Clock/1 -> Switch/2
  Gain1/1 -> [Q_set]
  Qset/1 -> Gain1/1
  [Q_abc] -> Gain3/1
  Gain3/1 -> Q/1
  [Q_abc] -> dVOC  - kappa=pi/2/5(q_m)
  Constant2/1 -> dVOC  - kappa=pi/2/4(v_m)
  dVOC  - kappa=pi/2/1(w_ref) -> [w]
  Constant1/1 -> dVOC  - kappa=pi/2/1(w_b)
  dVOC  - kappa=pi/2/2(theta_ref) -> [theta]
  [P_set] -> dVOC  - kappa=pi/2/3(p_set)
  [P_abc] -> dVOC  - kappa=pi/2/2(p_m)
  dVOC  - kappa=pi/2/3(v_ref_dq0) -> [v_ref_dq0]
  [Q_set] -> dVOC  - kappa=pi/2/6(q_set)
  Add4/1 -> LTI System3/1
  Add6/1 -> Gain16/1
  [P_s_abc] -> Add2/1
  [P_abc] -> Add2/2
  Gain16/1 -> Add4/1
  Constant3/1 -> Add6/1
  [P_set] -> Gain13/1
  Gain17/1 -> Add4/3
  Transfer Fcn2/1 -> Gain14/1
  Gain14/1 -> Add4/4
  [v_dc] -> Gain17/1
  Add2/1 -> Transfer Fcn2/1
  [v_dc] -> Add6/2
  Gain13/1 -> Add4/2
  connections:
  RL_c/RConn1 -- C_c1/LConn1 -- Current Measurement1/LConn1 -- Voltage Measurement4/LConn1
  C_c1/RConn1 -- Ground2/LConn1 -- C_a/RConn1 -- C_b/RConn1
  Universal Bridge/RConn2 -- i_dc1/LConn1 -- G_dc1/RConn1 -- C_dc1/RConn1 -- Voltage Measurement/LConn2
  Voltage Measurement1/LConn1 -- Current Measurement4/LConn1 -- Universal Bridge/LConn1
  Voltage Measurement2/LConn1 -- Current Measurement5/LConn1 -- Universal Bridge/LConn2
  Voltage Measurement3/LConn1 -- Universal Bridge/LConn3 -- Current Measurement6/LConn1
  Current Measurement1/RConn1 -- A/RConn1
  Current Measurement2/RConn1 -- B/RConn1
  Current Measurement3/RConn1 -- C/RConn1
  Voltage Measurement3/LConn2 -- Voltage Measurement1/LConn2 -- Voltage Measurement2/LConn2 -- Ground/LConn1
  Ground1/LConn1 -- Voltage Measurement4/LConn2 -- Voltage Measurement5/LConn2 -- Voltage Measurement6/LConn2
  Universal Bridge/RConn1 -- Voltage Measurement/LConn1 -- i_dc1/RConn1 -- G_dc1/LConn1 -- C_dc1/LConn1
  Current Measurement5/RConn1 -- RL_b/LConn1
  Current Measurement6/RConn1 -- RL_a/LConn1
  Current Measurement4/RConn1 -- RL_c/LConn1
  RL_a/RConn1 -- C_a/LConn1 -- Current Measurement3/LConn1 -- Voltage Measurement6/LConn1
  C_b/LConn1 -- Current Measurement2/LConn1 -- Voltage Measurement5/LConn1 -- RL_b/RConn1

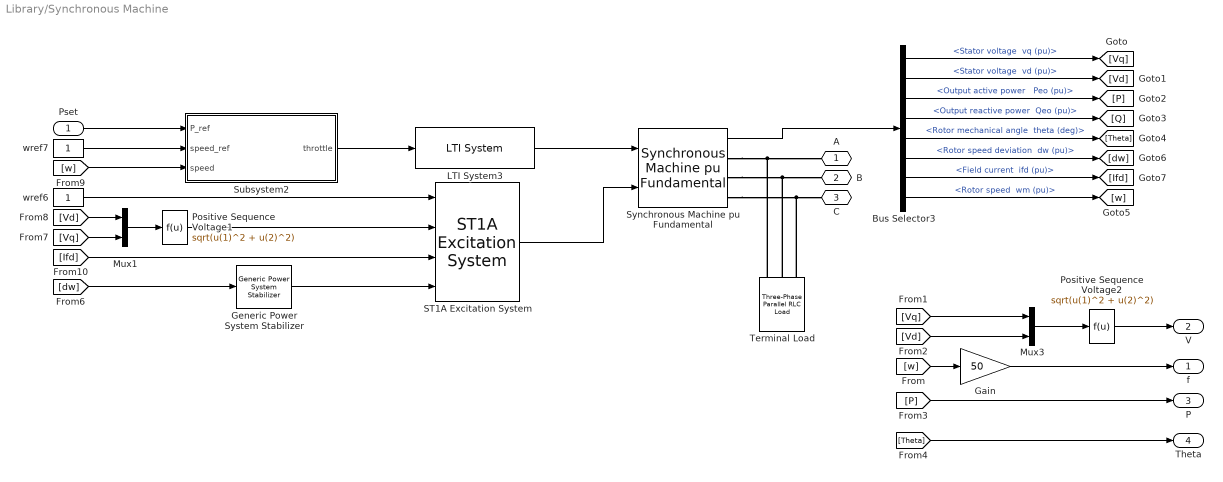
== system Library/Synchronous Machine ==
  Pset : Inport
  Bus Selector3 : BusSelector  OutputSignals="dq0 components.Stator voltage  vq (pu),dq0 components.Stator voltage  vd (pu),Output active power   Peo (pu),Output reactive power  Qeo (pu),Mechanical.Rotor mechanical angle  theta (deg),Mechanical.Rotor speed deviation  dw (pu),dq0 components.Field current  ifd (pu),Mechanical.Rotor speed  wm (pu)"
  Gain : Gain  Gain=50
  Generic Power System Stabilizer : powerlib/Machines/Generic Power System Stabilizer  Tsensor=30e-4  K=2.5  Twashout=2  Tleadlag1=[2*50e-3 0.01*20e-3]  Tleadlag2=[2*3 0.1*5.4]  VSlimits=2*[-0.15 0.15]  Vinit=0  Plot_On=off  MagdB_On=on  FreqRange=logspace(-2,2,500)
      settings: SourceProductName=Simscape Power Systems  SourceProductBaseCode=PS
  LTI System3 : cstblocks/LTI System  sys=tf(1,[tau_g 1])  IC=[]
  Mux1 : Mux  Inputs=2
  Mux3 : Mux  Inputs=2
  Positive Sequence Voltage1 : Fcn  Expr=sqrt(u(1)^2 + u(2)^2)
  Positive Sequence Voltage2 : Fcn  Expr=sqrt(u(1)^2 + u(2)^2)
  ST1A Excitation System : sps_avr/ST1A Excitation System  Tr=20e-4  KaTa=[210 0.001]  VIminmax=[-999 +999]  VAminmax=[-999 999]  VRminmax=[-6.0 6.43]  KfTf=[0.001 1]  TbTc=[0 0 0 0]  KLR=1  ILR=2  Kc=0.038  v0=[1 1]  TsBlock=0
      settings: SourceProductName=Simscape Power Systems  SourceProductBaseCode=PS
  Subsystem2 : Subsystem
  Synchronous Machine pu Fundamental : powerlib/Machines/Synchronous Machine pu Fundamental  PresetModel=No  MechanicalLoad=Mechanical power Pm  ShowDetailedParameters=on  RotorType=Salient-pole  Units=per unit fundamental parameters  MeasurementBus=off  NominalParameters="[100E6  V2_rms   50]"  Stator="[ 2.85E-03  0.114  1.19  0.36 ]"  Field="[ 5.79E-04  0.114]"  Dampers2=[0.0652, 0.5134, 0.0287, 0.2553, 7.765e-3, 0.9167 ]  Dampers1="[ 1.17E-02  0.182  1.97E-02  0.384 ]"  Mechanical=[ 3.7 0 20]  PolePairs=20  InitialConditions="[ 0  0  0  0  0  0  0  0  1 ]"  SetSaturation=off  Saturation=[0.6404,0.7127,0.8441,0.9214,0.9956,1.082,1.19,1.316,1.457;0.7,0.7698,0.8872,0.9466,0.9969,1.046,1.1,1.151,1.201]  LoadFlowParameters=[1,0,0,0,0]  TsPowergui=0  TsBlock=-1  IterativeModel=Trapezoidal non iterative  IterativeDiscreteModel=Trapezoidal non iterative  BusType=PV  Pref=0  Qref=0  Qmin=-inf  Qmax=inf  PLF=0  QLF=0
      settings: SourceProductName=Simscape Power Systems  SourceProductBaseCode=PS
  Terminal Load : powerlib/Elements/Three-Phase Parallel RLC Load  LConnTagsString=A|B|C  Configuration=Y (grounded)  NominalVoltage=V2_rms  Vabc=[1e3 1e3 1e3]  Vabcp=[1e3 1e3 1e3]  NominalFrequency=50  UnbalancedPower=off  ActivePower=1  InductivePower=0  CapacitivePower=0  Pabc=[10e3 9e3 11e3]  QLabc=[100 90 110]  QCabc=[100 90 110]  Pabcp=[10e3 9e3 11e3]  QLabcp=[100 90 110]  QCabcp=[100 90 110]  Measurements=None  LoadType=constant Z
  wref6 : Constant
  wref7 : Constant
  A : PMIOPort  Side=Right
  B : PMIOPort  Port=2  Side=Right
  C : PMIOPort  Port=3  Side=Right
  f : Outport
  V : Outport  Port=2
  P : Outport  Port=3
  Theta : Outport  Port=4
  wires:
  Gain/1 -> f/1
  Pset/1 -> Subsystem2/1(P_ref)
  Positive Sequence Voltage2/1 -> V/1
  wref7/1 -> Subsystem2/2(speed_ref)
  wref6/1 -> ST1A Excitation System/1
  Mux3/1 -> Positive Sequence Voltage2/1
  Synchronous Machine pu Fundamental/1 -> Bus Selector3/1
  [w] -> Gain/1
  [Vq] -> Mux3/1
  [Vd] -> Mux3/2
  [P] -> P/1
  [Theta] -> Theta/1
  [w] -> Subsystem2/3(speed)
  Subsystem2/1(throttle) -> LTI System3/1
  Bus Selector3/1 -> [Vq]  "<Stator voltage  vq (pu)>"
  Bus Selector3/2 -> [Vd]  "<Stator voltage  vd (pu)>"
  Bus Selector3/3 -> [P]  "<Output active power   Peo (pu)>"
  Bus Selector3/4 -> [Q]  "<Output reactive power  Qeo (pu)>"
  Bus Selector3/5 -> [Theta]  "<Rotor mechanical angle  theta (deg)>"
  Bus Selector3/6 -> [dw]  "<Rotor speed deviation  dw (pu)>"
  Bus Selector3/7 -> [Ifd]  "<Field current  ifd (pu)>"
  Bus Selector3/8 -> [w]  "<Rotor speed  wm (pu)>"
  LTI System3/1 -> Synchronous Machine pu Fundamental/1
  Generic Power System Stabilizer/1 -> ST1A Excitation System/4
  [dw] -> Generic Power System Stabilizer/1
  [Ifd] -> ST1A Excitation System/3
  Mux1/1 -> Positive Sequence Voltage1/1
  [Vd] -> Mux1/1
  [Vq] -> Mux1/2
  Positive Sequence Voltage1/1 -> ST1A Excitation System/2
  ST1A Excitation System/1 -> Synchronous Machine pu Fundamental/2
  connections:
  Terminal Load/LConn1 -- Synchronous Machine pu Fundamental/RConn1 -- A/RConn1
  Terminal Load/LConn3 -- Synchronous Machine pu Fundamental/RConn3 -- C/RConn1
  Terminal Load/LConn2 -- Synchronous Machine pu Fundamental/RConn2 -- B/RConn1

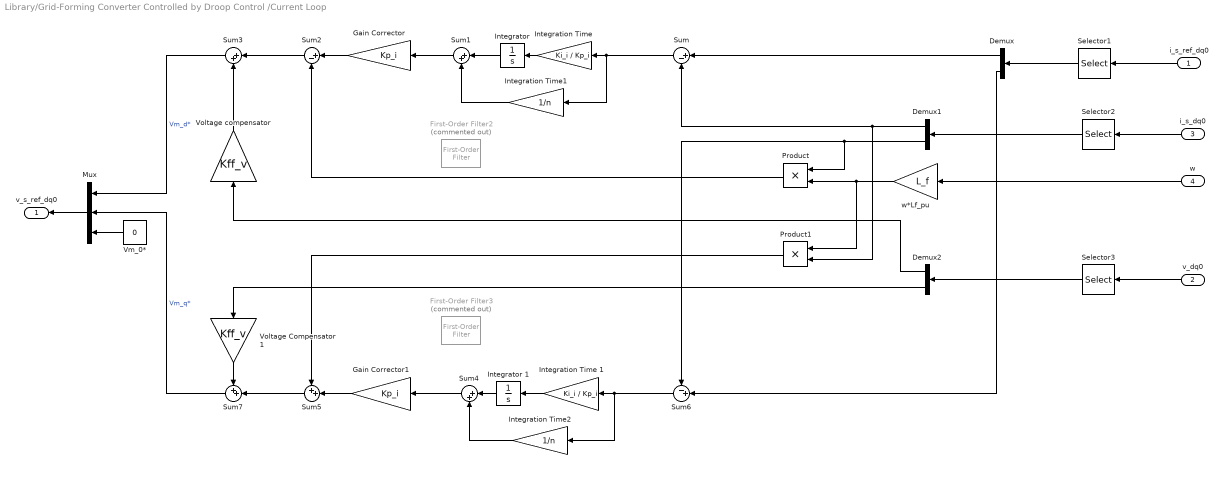
== system Library/Grid-Forming Converter Controlled by Droop Control /Current Loop ==
  i_s_ref_dq0 : Inport
  v_dq0 : Inport  Port=2
  i_s_dq0 : Inport  Port=3
  w : Inport  Port=4
  Demux : Demux  Outputs=2
  Demux1 : Demux  Outputs=2
  Demux2 : Demux  Outputs=2
  First-Order Filter2 : powerlib_meascontrol/Filters/First-Order Filter  Commented=on  FilterType=Lowpass  Tc=25e-3  Ts=0  Initialize=on  Vac_Init=[0, 0, 50]  Vdc_Init=1  PlotResponse=off  FreqRange="[0,  200,  1]"
      settings: SourceProductName=Simscape Power Systems
  First-Order Filter3 : powerlib_meascontrol/Filters/First-Order Filter  Commented=on  FilterType=Lowpass  Tc=25e-3  Ts=0  Initialize=on  Vac_Init=[0, 0, 50]  Vdc_Init=0  PlotResponse=off  FreqRange="[0,  200,  1]"
      settings: SourceProductName=Simscape Power Systems
  Gain Corrector : Gain  Gain=Kp_i
  Gain Corrector1 : Gain  Gain=Kp_i
  Integration Time : Gain  Gain=Ki_i / Kp_i
  Integration Time 1 : Gain  Gain=Ki_i / Kp_i
  Integration Time1 : Gain  Gain=1/n
  Integration Time2 : Gain  Gain=1/n
  Integrator : Integrator  InitialCondition=0.0001
  Integrator 1 : Integrator
  Mux : Mux  Inputs=3
  Product : Product  RndMeth=Zero
  Product1 : Product  RndMeth=Zero
  Selector1 : Selector  InputPortWidth=3  IndexOptions=Index vector (dialog)  Indices=[1 2]  OutputSizes=1
  Selector2 : Selector  InputPortWidth=3  IndexOptions=Index vector (dialog)  Indices=[1 2]  OutputSizes=1
  Selector3 : Selector  InputPortWidth=3  IndexOptions=Index vector (dialog)  Indices=[1 2]  OutputSizes=1
  Sum : Sum  Inputs=|+-
  Sum1 : Sum  Inputs=|++
  Sum2 : Sum  Inputs=|+-
  Sum3 : Sum  Inputs=|++
  Sum4 : Sum  Inputs=|++
  Sum5 : Sum  Inputs=++|
  Sum6 : Sum  Inputs=-+|
  Sum7 : Sum  Inputs=++|
  Vm_0* : Constant  Value=0
  Voltage Compensator 1 : Gain  Gain=Kff_v
  Voltage compensator : Gain  Gain=Kff_v
  w*Lf_pu : Gain  Gain=L_f
  v_s_ref_dq0 : Outport
  wires:
  Sum/1 -> Integration Time/1, Integration Time1/1
  Integration Time 1/1 -> Integrator 1/1
  Integration Time/1 -> Integrator/1
  Sum5/1 -> Sum7/2
  Sum6/1 -> Integration Time 1/1, Integration Time2/1
  Demux/1 -> Sum/1
  Sum3/1 -> Mux/1  "Vm_d*"
  Sum7/1 -> Mux/2  "Vm_q*"
  Demux2/2 -> Voltage Compensator 1/1
  Voltage Compensator 1/1 -> Sum7/1
  Product/1 -> Sum2/2
  w*Lf_pu/1 -> Product1/1, Product/2
  i_s_ref_dq0/1 -> Selector1/1
  v_dq0/1 -> Selector3/1
  Integrator 1/1 -> Sum4/1
  Voltage compensator/1 -> Sum3/2
  Sum1/1 -> Gain Corrector/1
  Sum2/1 -> Sum3/1
  Sum4/1 -> Gain Corrector1/1
  Demux/2 -> Sum6/2
  Selector1/1 -> Demux/1
  Gain Corrector/1 -> Sum2/1
  w/1 -> w*Lf_pu/1
  Mux/1 -> v_s_ref_dq0/1
  Selector2/1 -> Demux1/1
  i_s_dq0/1 -> Selector2/1
  Selector3/1 -> Demux2/1
  Demux1/2 -> Product/1, Sum6/1
  Vm_0*/1 -> Mux/3
  Integrator/1 -> Sum1/1
  Demux1/1 -> Product1/2, Sum/2
  Demux2/1 -> Voltage compensator/1
  Product1/1 -> Sum5/1
  Gain Corrector1/1 -> Sum5/2
  Integration Time1/1 -> Sum1/2
  Integration Time2/1 -> Sum4/2
